simulink model "integrators"  (R2022b)
settings: Solver=VariableStepAuto  StartTime=0.0  StopTime=10.0  RelTol=1e-3
undefined symbols (not defined in the file): DiscIntNeverNeededParam
settings Model: Creator=yasso  LastModifiedBy=yasso

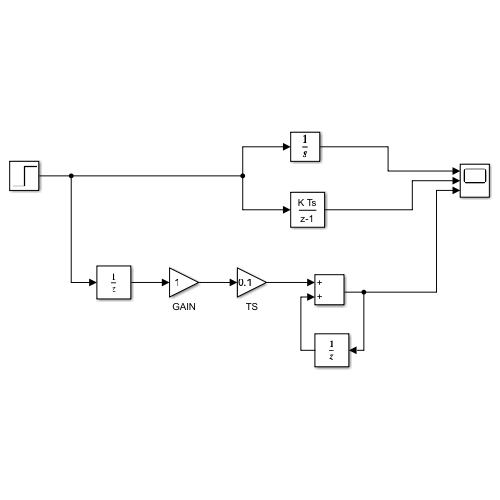
[thumbnail: Simulink's stored preview of the top-level diagram]
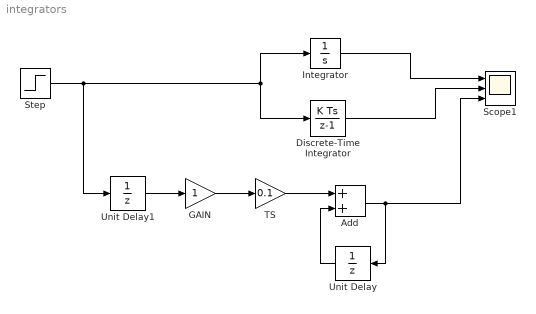
== system integrators ==
  Add : Sum
  Discrete-Time Integrator : DiscreteIntegrator  SampleTime=-1  ICPrevOutput=DiscIntNeverNeededParam  ICPrevScaledInput=DiscIntNeverNeededParam
  GAIN : Gain
  Integrator : Integrator
  Scope1 : Scope  NumInputPorts=3
  Step : Step  SampleTime=0
  TS : Gain  Gain=0.1
  Unit Delay : UnitDelay  SampleTime=-1  HasFrameUpgradeWarning=on
  Unit Delay1 : UnitDelay  SampleTime=-1  HasFrameUpgradeWarning=on
  wires:
  Add/1 -> Unit Delay/1, Scope1/3
  Unit Delay/1 -> Add/2
  GAIN/1 -> TS/1
  TS/1 -> Add/1
  Integrator/1 -> Scope1/1
  Step/1 -> Discrete-Time Integrator/1, Integrator/1, Unit Delay1/1
  Discrete-Time Integrator/1 -> Scope1/2
  Unit Delay1/1 -> GAIN/1
